simulink model "Smart_City_QCar2_self_driving_stack_r2020a"  (R2020a)
settings: Solver=ode1  StartTime=0.0  StopTime=inf  FixedStep=Controller_Sample_Time  RelTol=1e-3  EnableMultiTasking=on
undefined symbols (not defined in the file): angles_qcar2, Audio_Sample_Time, cal_pos, cameraStepSize, Cobra_Start, Controller_Sample_Time, CSI_Sample_Time, DiscIntNeverNeededParam, engine, gcbh, GyroKF_P0, GyroKF_Q, GyroKF_R, GyroKF_X0, height, HIL, honk, ImageDisplay_Sample_Time, Initialization_Time, Joystick_Sample_Time, JPEG, left, LiDAR_Sample_Time, map_mask, NN_Sample_Time, path_x, path_x2, path_x3, path_x4, path_x5, path_x6, path_x7, path_y, path_y2, path_y3, path_y4, path_y5, path_y6, path_y7, Point, put_me_down, qc_get_step_size, qcar2_lidar_to_map_rotation, QCarEKF_L, QCarEKF_P0, QCarEKF_Q, QCarEKF_R_combined, QCarEKF_R_heading, QcarKF_X0, range_qcar2, RealSense_Sample_Time, top, truck_start, video_display_show, width
libraries: quarc_library x65, simulink_extras x12, simulink x8
(part 2 of 4)

== system Smart_City_QCar2_self_driving_stack_r2020a/Rate Timing Plots/monitorTiming1 ==
  note: moniorTiming Module:
      |
      | This subsystem outputs the sample time and computation time of the model.
      |
      | Outputs:
      | sampleTime (s) n/a : Sample time (unfiltered and filtered) in seconds.
      | computationTime (s) n/a : Computation time (unfiltered and filtered) in seconds.
      |
      | Usage:
      | Compare the Sample Time (s) output to a constant (qc_get_step_size) to monitor whether or not the desired sample time is being achieved. The Computation Time (s) values should be lower than the corresponding sample time value to ensure that the solver has enough time per time step.
  note: Timing Performance
  Computation Time : quarc_library/Sources/Time/Computation Time  sample_time=qc_get_step_size  use_model=on  use_cpu_time=off
  Constant : Constant  Value=qc_get_step_size  SampleTime=-1
  Mux : Mux  Inputs=3
  Sample Time : quarc_library/Sources/Time/Sample Time  Priority=-99  sample_time=qc_get_step_size
  Timing (s) : Outport  VectorParamsAs1DForOutWhenUnconnected=off
  wires:
  Constant/1 -> Mux/2
  Sample Time/1 -> Mux/1
  Mux/1 -> Timing (s)/1
  Computation Time/1 -> Mux/3

== system Smart_City_QCar2_self_driving_stack_r2020a/Rate Timing Plots/monitorTiming2 ==
  note: moniorTiming Module:
      |
      | This subsystem outputs the sample time and computation time of the model.
      |
      | Outputs:
      | sampleTime (s) n/a : Sample time (unfiltered and filtered) in seconds.
      | computationTime (s) n/a : Computation time (unfiltered and filtered) in seconds.
      |
      | Usage:
      | Compare the Sample Time (s) output to a constant (qc_get_step_size) to monitor whether or not the desired sample time is being achieved. The Computation Time (s) values should be lower than the corresponding sample time value to ensure that the solver has enough time per time step.
  note: Timing Performance
  Computation Time : quarc_library/Sources/Time/Computation Time  sample_time=RealSense_Sample_Time  use_model=on  use_cpu_time=off
  Constant : Constant  Value=RealSense_Sample_Time  SampleTime=-1
  Mux : Mux  Inputs=3
  Sample Time : quarc_library/Sources/Time/Sample Time  Priority=-99  sample_time=RealSense_Sample_Time
  Timing (s) : Outport  VectorParamsAs1DForOutWhenUnconnected=off
  wires:
  Constant/1 -> Mux/2
  Sample Time/1 -> Mux/1
  Mux/1 -> Timing (s)/1
  Computation Time/1 -> Mux/3

== system Smart_City_QCar2_self_driving_stack_r2020a/Rate Timing Plots/monitorTiming3 ==
  note: Timing Performance
  note: moniorTiming Module:
      |
      | This subsystem outputs the sample time and computation time of the model.
      |
      | Outputs:
      | sampleTime (s) n/a : Sample time (unfiltered and filtered) in seconds.
      | computationTime (s) n/a : Computation time (unfiltered and filtered) in seconds.
      |
      | Usage:
      | Compare the Sample Time (s) output to a constant (qc_get_step_size) to monitor whether or not the desired sample time is being achieved. The Computation Time (s) values should be lower than the corresponding sample time value to ensure that the solver has enough time per time step.
  Computation Time : quarc_library/Sources/Time/Computation Time  sample_time=ImageDisplay_Sample_Time  use_model=on  use_cpu_time=off
  Constant : Constant  Value=ImageDisplay_Sample_Time  SampleTime=-1
  Mux : Mux  Inputs=3
  Sample Time : quarc_library/Sources/Time/Sample Time  Priority=-99  sample_time=ImageDisplay_Sample_Time
  Timing (s) : Outport  VectorParamsAs1DForOutWhenUnconnected=off
  wires:
  Computation Time/1 -> Mux/3
  Mux/1 -> Timing (s)/1
  Sample Time/1 -> Mux/1
  Constant/1 -> Mux/2

== system Smart_City_QCar2_self_driving_stack_r2020a/Rate Timing Plots/monitorTiming4 ==
  note: Timing Performance
  note: moniorTiming Module:
      |
      | This subsystem outputs the sample time and computation time of the model.
      |
      | Outputs:
      | sampleTime (s) n/a : Sample time (unfiltered and filtered) in seconds.
      | computationTime (s) n/a : Computation time (unfiltered and filtered) in seconds.
      |
      | Usage:
      | Compare the Sample Time (s) output to a constant (qc_get_step_size) to monitor whether or not the desired sample time is being achieved. The Computation Time (s) values should be lower than the corresponding sample time value to ensure that the solver has enough time per time step.
  Computation Time : quarc_library/Sources/Time/Computation Time  sample_time=Joystick_Sample_Time  use_model=on  use_cpu_time=off
  Constant : Constant  Value=Joystick_Sample_Time  SampleTime=-1
  Mux : Mux  Inputs=3
  Sample Time : quarc_library/Sources/Time/Sample Time  Priority=-99  sample_time=Joystick_Sample_Time
  Timing (s) : Outport  VectorParamsAs1DForOutWhenUnconnected=off
  wires:
  Computation Time/1 -> Mux/3
  Mux/1 -> Timing (s)/1
  Sample Time/1 -> Mux/1
  Constant/1 -> Mux/2

== system Smart_City_QCar2_self_driving_stack_r2020a/Rate Timing Plots/monitorTiming5 ==
  note: moniorTiming Module:
      |
      | This subsystem outputs the sample time and computation time of the model.
      |
      | Outputs:
      | sampleTime (s) n/a : Sample time (unfiltered and filtered) in seconds.
      | computationTime (s) n/a : Computation time (unfiltered and filtered) in seconds.
      |
      | Usage:
      | Compare the Sample Time (s) output to a constant (qc_get_step_size) to monitor whether or not the desired sample time is being achieved. The Computation Time (s) values should be lower than the corresponding sample time value to ensure that the solver has enough time per time step.
  note: Timing Performance
  Computation Time : quarc_library/Sources/Time/Computation Time  sample_time=LiDAR_Sample_Time  use_model=on  use_cpu_time=off
  Constant : Constant  Value=LiDAR_Sample_Time  SampleTime=-1
  Mux : Mux  Inputs=3
  Sample Time : quarc_library/Sources/Time/Sample Time  Priority=-99  sample_time=LiDAR_Sample_Time
  Timing (s) : Outport  VectorParamsAs1DForOutWhenUnconnected=off
  wires:
  Constant/1 -> Mux/2
  Sample Time/1 -> Mux/1
  Mux/1 -> Timing (s)/1
  Computation Time/1 -> Mux/3

== system Smart_City_QCar2_self_driving_stack_r2020a/Rate Timing Plots/monitorTiming6 ==
  note: Timing Performance
  note: moniorTiming Module:
      |
      | This subsystem outputs the sample time and computation time of the model.
      |
      | Outputs:
      | sampleTime (s) n/a : Sample time (unfiltered and filtered) in seconds.
      | computationTime (s) n/a : Computation time (unfiltered and filtered) in seconds.
      |
      | Usage:
      | Compare the Sample Time (s) output to a constant (qc_get_step_size) to monitor whether or not the desired sample time is being achieved. The Computation Time (s) values should be lower than the corresponding sample time value to ensure that the solver has enough time per time step.
  Computation Time : quarc_library/Sources/Time/Computation Time  sample_time=NN_Sample_Time  use_model=on  use_cpu_time=off
  Constant : Constant  Value=NN_Sample_Time  SampleTime=-1
  Mux : Mux  Inputs=3
  Sample Time : quarc_library/Sources/Time/Sample Time  Priority=-99  sample_time=NN_Sample_Time
  Timing (s) : Outport  VectorParamsAs1DForOutWhenUnconnected=off
  wires:
  Computation Time/1 -> Mux/3
  Mux/1 -> Timing (s)/1
  Sample Time/1 -> Mux/1
  Constant/1 -> Mux/2

== system Smart_City_QCar2_self_driving_stack_r2020a/Rate Timing Plots/monitorTiming7 ==
  note: Timing Performance
  note: moniorTiming Module:
      |
      | This subsystem outputs the sample time and computation time of the model.
      |
      | Outputs:
      | sampleTime (s) n/a : Sample time (unfiltered and filtered) in seconds.
      | computationTime (s) n/a : Computation time (unfiltered and filtered) in seconds.
      |
      | Usage:
      | Compare the Sample Time (s) output to a constant (qc_get_step_size) to monitor whether or not the desired sample time is being achieved. The Computation Time (s) values should be lower than the corresponding sample time value to ensure that the solver has enough time per time step.
  Computation Time : quarc_library/Sources/Time/Computation Time  sample_time=1  use_model=on  use_cpu_time=off
  Constant : Constant  SampleTime=-1
  Mux : Mux  Inputs=3
  Sample Time : quarc_library/Sources/Time/Sample Time  Priority=-99  sample_time=1
  Timing (s) : Outport  VectorParamsAs1DForOutWhenUnconnected=off
  wires:
  Computation Time/1 -> Mux/3
  Mux/1 -> Timing (s)/1
  Sample Time/1 -> Mux/1
  Constant/1 -> Mux/2

== system Smart_City_QCar2_self_driving_stack_r2020a/Rate Timing Plots/monitorTiming8 ==
  note: moniorTiming Module:
      |
      | This subsystem outputs the sample time and computation time of the model.
      |
      | Outputs:
      | sampleTime (s) n/a : Sample time (unfiltered and filtered) in seconds.
      | computationTime (s) n/a : Computation time (unfiltered and filtered) in seconds.
      |
      | Usage:
      | Compare the Sample Time (s) output to a constant (qc_get_step_size) to monitor whether or not the desired sample time is being achieved. The Computation Time (s) values should be lower than the corresponding sample time value to ensure that the solver has enough time per time step.
  note: Timing Performance
  Computation Time : quarc_library/Sources/Time/Computation Time  sample_time=Audio_Sample_Time  use_model=on  use_cpu_time=off
  Constant : Constant  Value=Audio_Sample_Time  SampleTime=-1
  Mux : Mux  Inputs=3
  Sample Time : quarc_library/Sources/Time/Sample Time  Priority=-99  sample_time=Audio_Sample_Time
  Timing (s) : Outport  VectorParamsAs1DForOutWhenUnconnected=off
  wires:
  Constant/1 -> Mux/2
  Sample Time/1 -> Mux/1
  Mux/1 -> Timing (s)/1
  Computation Time/1 -> Mux/3

== system Smart_City_QCar2_self_driving_stack_r2020a/RealSense Camera/Newer Depth ==
  In1 : Inport
  Channel : quarc_library/Signal Routing/Channel  channel=0  buffer_size=1
  Image Compress : quarc_library/Image Processing/Generic/Image Compress  algorithm=JPEG  source=Internal dialog parameter  quality=quality  output_dim=-1
  Video Display : quarc_library/Multimedia/Video Display  Tag=Smart_City_QCar2_self_driving_stack_r2020a/RealSense Camera/Newer Depth/Video Display  sample_time=sample_time  use_hardware=on
  wires:
  Image Compress/1 -> Channel/1
  In1/1 -> Image Compress/1
  Channel/1 -> Video Display/1

== system Smart_City_QCar2_self_driving_stack_r2020a/RealSense Camera/RealSense Capture ==
  AND : Logic  Commented=on  AllPortsSameDT=off  OutDataTypeStr=boolean
  AND1 : Logic  Commented=on  IconShape=distinctive  AllPortsSameDT=off  OutDataTypeStr=boolean
  Compare To Constant : simulink/Logic and Bit Operations/Compare To Constant  Commented=on  relop===  const=2  OutDataTypeStr=boolean
  Compare To Constant1 : simulink/Logic and Bit Operations/Compare To Constant  Commented=on  relop=>=  const=0  OutDataTypeStr=boolean
  Constant : Constant  Commented=on  Value=[1 0 0 0 0]
  Display : Display  Commented=on
  Display1 : Display  Commented=on
  Display2 : Display  Commented=on
  Image Compress : quarc_library/Image Processing/Generic/Image Compress  Commented=on  algorithm=JPEG  source=Internal dialog parameter  quality=50  output_dim=-1
  Image Filter : quarc_library/Image Processing/Generic/Image Filter  filter_type=Depth hole-fill  source_of_roi=Internal dialog parameter  roi_style=[top, left, height, width]  roi=[]  maximum_roi=[]  roi_zone=Operate inside region of interest  border_type=Replicate  border_value=[0 0 0]  kernel_size=5  sigma=10  mask_size=[3 3]  kernel=int16([-2 -1 0; -1 1 1; 0 1 2])  divisor=1  offset=0  rounding=Nearest  algorithm_hint=None  threshold=100  alpha=0.9  num_frames=8  num_valid=1  gap_threshold=10  depth_threshold=255  iterations=2  norm_type=L1
      settings: AttributesFormatString=(%<filter_type>)  SourceProductName=QUARC Targets
  Image Filter1 : quarc_library/Image Processing/Generic/Image Filter  filter_type=Depth temporal low-pass  source_of_roi=Internal dialog parameter  roi_style=[top, left, height, width]  roi=[]  maximum_roi=[]  roi_zone=Operate inside region of interest  border_type=Replicate  border_value=[0 0 0]  kernel_size=5  sigma=10  mask_size=[3 3]  kernel=int16([-2 -1 0; -1 1 1; 0 1 2])  divisor=1  offset=0  rounding=Nearest  algorithm_hint=None  threshold=100  alpha=0.9  num_frames=4  num_valid=1  gap_threshold=10  depth_threshold=255  iterations=2  norm_type=L1
      settings: AttributesFormatString=(%<filter_type>)  SourceProductName=QUARC Targets
  Memory : Memory  Commented=on  InheritSampleTime=on
  NN New : Scope  Commented=on
  NN Receive : Scope  Commented=on
  Rate Transition : RateTransition  Commented=on  OutPortSampleTime=NN_Sample_Time
  Scope : Scope
  Stream Server : quarc_library/Communications/Basic/Stream Server  Commented=on  uri_source=Specify via dialog (do not evaluate)  uri=tcpip://remotehost:18999  send_buffer_size=640*360*3  receive_buffer_size=6*32  byte_order=little endian (Intel - LSB first)  optimization=Minimum latency  send_options=Send most recent data  receive_options=Receive most recent data  default_value=zeros(1,5,'single')  sample_time=NN_Sample_Time  active=off  implementation=Use blocking I/O in a separate thread  send_fifo_size=2  receive_fifo_size=2  send_priority=0  receive_priority=0  send_dimensions=on  receive_dimensions=off  max_dimensions=-1  data_type=single  type_expr=BusObject
      settings: AttributesFormatString="\"tcpip://remotehost:18999\""
  Switch : Switch  Commented=on  Criteria=u2 > Threshold  Threshold=0.5
  Terminator{,1..4} (5 alike) : Terminator
  Terminator5 : Terminator  Commented=on
  Video3D Capture : quarc_library/Multimedia/Video3D Capture  object_name=RealSense  stream_type=Depth  stream_index=0  resolution=640 x 360  width=640  height=360  output_format=Distance in meters (HxW)  data_type=single  sample_time=RealSense_Sample_Time  camera_intrinsics=off  depth_scale=off  brightness_override=Do not override  brightness=50.0  contrast_override=Do not override  contrast=50.0  hue_override=Do not override  hue=50.0  saturation_override=Do not override  saturation=50.0  sharpness_override=Do not override  sharpness=50.0  gamma_override=Do not override  gamma=50.0  gain_override=Do not override  gain=50.0  backlightcompensation_override=Do not override  backlightcompensation=50.0  whitebalance_override=Automatic white balance  whitebalance=50.0  exposure_override=Automatic exposure  exposure=30.0  emitter=Enable laser emitter  preset=Do not set camera presets
  Video3D Capture1 : quarc_library/Multimedia/Video3D Capture  object_name=RealSense  stream_type=RGB  stream_index=0  resolution=1920 x 1080  width=1920  height=1080  output_format=MATLAB RGB (HxWx3)  data_type=uint8  sample_time=RealSense_Sample_Time*1  camera_intrinsics=off  depth_scale=off  brightness_override=Do not override  brightness=50.0  contrast_override=Do not override  contrast=50.0  hue_override=Do not override  hue=50.0  saturation_override=Do not override  saturation=50.0  sharpness_override=Do not override  sharpness=50.0  gamma_override=Do not override  gamma=50.0  gain_override=Do not override  gain=50.0  backlightcompensation_override=Do not override  backlightcompensation=50.0  whitebalance_override=Automatic white balance  whitebalance=50.0  exposure_override=Automatic exposure  exposure=30.0  emitter=Enable laser emitter  preset=Do not set camera presets
  Video3D Initialize : quarc_library/Multimedia/Video3D Initialize  object_name=RealSense  source=Device  identifier=0  file=sample.bag  sample_time=RealSense_Sample_Time  active=on
  New : Outport
  Depth Image : Outport  Port=2
  Sign Probabilities : Outport  Port=3
  wires:
  Video3D Capture/4 -> New/1
  Video3D Capture/2 -> Terminator4/1
  Video3D Capture/3 -> Terminator3/1
  Video3D Capture/1 -> Image Filter/1
  Video3D Initialize/1 -> Terminator/1
  Switch/1 -> Sign Probabilities/1
  Video3D Capture1/1 -> Rate Transition/1
  Constant/1 -> Switch/3
  Compare To Constant1/1 -> AND/2
  Stream Server/4 -> NN Receive/1, Switch/1
  Stream Server/2 -> Compare To Constant1/1, Display1/1
  Stream Server/5 -> NN New/1, Switch/2
  Stream Server/3 -> Terminator5/1
  Compare To Constant/1 -> AND/1
  Video3D Capture1/2 -> Terminator1/1
  Video3D Capture1/3 -> Terminator2/1
  Stream Server/1 -> Compare To Constant/1, Display/1
  Memory/1 -> AND1/2
  AND/1 -> Display2/1, Memory/1
  Video3D Capture1/4 -> Scope/1, AND1/1
  AND1/1 -> Stream Server/2
  Rate Transition/1 -> Image Compress/1
  Image Compress/1 -> Stream Server/1
  Image Filter/1 -> Image Filter1/1
  Image Filter1/1 -> Depth Image/1

== system Smart_City_QCar2_self_driving_stack_r2020a/RealSense Camera/obstacleDetection Markham March 22 ==
  note: %
  note: m
  note: m
  note: %
  note: px
  note: px
  note: %
  note: %
  imageDepth : Inport
  steering (rad) : Inport  Port=2
  Enable : EnablePort  PropagateVarSize=During execution
  Add : Sum
  Bias : Constant  Value=0
  Box Color : Constant  Value=[255 0 0]
  Constant1 : Constant  Value=200
  Constant2 : Constant  Value=.15
  Constant3 : Constant
  Constant4 : Constant  Value=50
  Constant5 : Constant  Value=0.5
  Constant6 : Constant  Value=0.5
  Constant7 : Constant  Value=0.6
  Constant8 : Constant  Value=0.6
  Display : Display
  Draw Lines Module : MATLAB Function  TreatAsAtomicUnit=on
  Image Convert : quarc_library/Image Processing/Generic/Image Convert  input_format=MATLAB greyscale (HxW)  padding=0  output_format=MATLAB greyscale (HxW)  data_type=uint16
      settings: AttributesFormatString=(%<input_format>)  SourceProductName=QUARC Targets
  Saturation : Saturate  UpperLimit=2  LowerLimit=0.05
  Saturation1 : Saturate  UpperLimit=1  LowerLimit=0
  Scope : Scope
  Steering based image subselector : MATLAB Function  TreatAsAtomicUnit=on
  max white for 8m : Gain  Gain=1/2.5
  imageDepthForDisplay : Outport  VectorParamsAs1DForOutWhenUnconnected=off
  distance (m) : Outport  Port=2  VectorParamsAs1DForOutWhenUnconnected=off
  wires:
  Saturation1/1 -> Image Convert/1
  Constant6/1 -> Steering based image subselector/8(maxSteering)
  Steering based image subselector/2(distance) -> Add/1, Scope/1
  Constant5/1 -> Steering based image subselector/7(vertCenter)
  Constant4/1 -> Steering based image subselector/6(height)
  Constant1/1 -> Steering based image subselector/5(width)
  Constant3/1 -> Steering based image subselector/4(maxDistance)
  Constant2/1 -> Steering based image subselector/3(minDistance)
  steering (rad)/1 -> Steering based image subselector/2(steering)
  Draw Lines Module/1(img_out) -> imageDepthForDisplay/1
  Steering based image subselector/1(pts) -> Draw Lines Module/2(pts)
  Image Convert/1 -> Draw Lines Module/1(img_in)
  max white for 8m/1 -> Saturation1/1
  imageDepth/1 -> Steering based image subselector/1(depth), max white for 8m/1
  Bias/1 -> Add/2
  Add/1 -> Saturation/1, Display/1
  Saturation/1 -> distance (m)/1
  Box Color/1 -> Draw Lines Module/3(color)
  Constant7/1 -> Steering based image subselector/9(reduction)
  Constant8/1 -> Steering based image subselector/10(maxSteeringWidth)

== system Smart_City_QCar2_self_driving_stack_r2020a/Speed & Steering Commander/Cross Track Controller ==
  closest point : Inport
  distance : Inport  Port=2
  xy : Inport  Port=3
  Heading : Inport  Port=4
  Commanded_Speed : Inport  Port=5
  Path : Inport  Port=6
  Constant : Constant  Value=0
  Constant1 : Constant
  Constant6 : Constant  Value=Initialization_Time
  Cos : Trigonometry  Operator=cos
  Cos1 : Trigonometry
  Cross Product : quarc_library/Math Operations/Vectors/Cross Product
      settings: SourceProductName=QUARC Targets
  Demux : Demux  Outputs=3
  Equal : RelationalOperator  Operator===  OutDataTypeStr=boolean  RndMeth=Simplest
  Equal1 : RelationalOperator  Operator=~=  OutDataTypeStr=boolean  RndMeth=Simplest
  Gain3 : Gain
  Gain6 : Gain  Gain=3
  GreaterThan : RelationalOperator  Operator=<  OutDataTypeStr=boolean  RndMeth=Simplest
  Integrator : Integrator  ExternalReset=level  LimitOutput=on  UpperSaturationLimit=.2  LowerSaturationLimit=-.2
  Integrator1 : Integrator  ExternalReset=level  LimitOutput=on  UpperSaturationLimit=1  LowerSaturationLimit=0
  Memory1 : Memory  InitialCondition=6  InheritSampleTime=on  LinearizeMemory=on  LinearizeAsDelay=on
  Mux : Mux  Inputs=3
  Mux1 : Mux  Inputs=2
  Mux2 : Mux  Inputs=2
  OR : Logic  Operator=OR  Inputs=3  IconShape=distinctive  AllPortsSameDT=off  OutDataTypeStr=boolean
  Product : Product
  Product3 : Product
  Radians to Degrees : simulink_extras/Transformations/Radians to Degrees
  Saturation1 : Saturate  UpperLimit=.2  LowerLimit=-.2
  Scope1 : Scope  NumInputPorts=2
  Sign : Signum
  Sum : Sum  Inputs=+-
  Sum2 : Sum
  Time1 : quarc_library/Sources/Time/Time  time_source=Wall clock  sample_time=qc_get_step_size
  steering correction : Outport
  wires:
  Heading/1 -> Cos1/1, Cos/1
  Cos/1 -> Mux/1
  Cos1/1 -> Mux/2
  xy/1 -> Sum/2
  closest point/1 -> Sum/1
  Sum/1 -> Mux1/1
  Mux1/1 -> Cross Product/2
  Mux/1 -> Cross Product/1
  Cross Product/1 -> Demux/1
  Demux/3 -> Sign/1
  Sign/1 -> Product3/1
  Gain6/1 -> Integrator/1
  Product3/1 -> Gain3/1, Gain6/1
  Integrator/1 -> Mux2/1, Sum2/1
  Saturation1/1 -> Mux2/2, Sum2/2
  distance/1 -> Product3/2
  Sum2/1 -> steering correction/1
  Commanded_Speed/1 -> Equal/1
  Constant/1 -> Equal/2
  Path/1 -> Equal1/2, Memory1/1
  Memory1/1 -> Equal1/1
  Equal1/1 -> OR/2
  Equal/1 -> OR/1
  OR/1 -> Scope1/1, Integrator1/2, Integrator/2
  Constant1/1 -> Integrator1/1
  Product/1 -> Saturation1/1
  Gain3/1 -> Product/1
  Integrator1/1 -> Product/2
  Mux2/1 -> Radians to Degrees/1
  Radians to Degrees/1 -> Scope1/2
  Time1/1 -> GreaterThan/1
  Constant6/1 -> GreaterThan/2
  GreaterThan/1 -> OR/3

== system Smart_City_QCar2_self_driving_stack_r2020a/Speed & Steering Commander/Infrastructure Car Detection Speed Adjust ==
  obstacleDistance (m) : Inport
  Desired Speed Command : Inport  Port=2
  Constant : Constant  Value=0.3
  Constant1 : Constant  Value=.4
  Constant2 : Constant
  Less Than : RelationalOperator  Operator=<  OutDataTypeStr=boolean  RndMeth=Simplest
  MATLAB Function : MATLAB Function  TreatAsAtomicUnit=on
  Scope : Scope  NumInputPorts=2
  Adjusted Speed Command : Outport  VectorParamsAs1DForOutWhenUnconnected=off
  Honk : Outport  Port=2
  wires:
  Desired Speed Command/1 -> MATLAB Function/4(nominal_speed)
  MATLAB Function/1(speed_cmd) -> Adjusted Speed Command/1, Scope/1
  Less Than/1 -> Honk/1
  Constant1/1 -> Less Than/2
  obstacleDistance (m)/1 -> MATLAB Function/1(obstacle_distance), Scope/2, Less Than/1
  Constant/1 -> MATLAB Function/2(stop_distance)  "stop distance (m)"
  Constant2/1 -> MATLAB Function/3(nominal_tracking_distance)  "nominal tracking distance (m)"

== system Smart_City_QCar2_self_driving_stack_r2020a/Speed & Steering Commander/Path Commander ==
  note: Tunable
      | Params
  note: Changed the abs and the duration
  path : Inport
  xy : Inport  Port=2
  look_ahead_d : Inport  Port=3
  Data Type Conversion : DataTypeConversion
  Display : Display
  "Distance  " : Scope
  Distance (m) to a viable path : Constant  Value=0.05
  Duration that car is within distance of viable path : Constant  Value=0.2
  Less Than Threshold : Subsystem
  Multiport Switch : MultiPortSwitch  Inputs=7  DiagnosticForDefault=None
  Multiport Switch1 : MultiPortSwitch  Inputs=7  DiagnosticForDefault=None
  Multiport Switch2 : MultiPortSwitch  Inputs=7  DiagnosticForDefault=None
  Mux : Mux  Inputs=7
  Path 1  Look Ahead Generator : Subsystem
  Path 2  Look Ahead Generator : Subsystem
  Path 3  Look Ahead Generator : Subsystem
  Path 4  Look Ahead Generator : Subsystem
  Path 5  Look Ahead Generator : Subsystem
  Path 6  Look Ahead Generator : Subsystem
  Path 7  Look Ahead Generator : Subsystem
  Turn Paths on and Off : Gain  Gain=map_mask
  xy_cmd : Outport
  Path_Options : Outport  Port=2
  closest point : Outport  Port=3
  distance : Outport  Port=4
  wires:
  look_ahead_d/1 -> Path 7  Look Ahead Generator/2(look_ahead_d), Path 6  Look Ahead Generator/2(look_ahead_d), Path 5  Look Ahead Generator/2(look_ahead_d), Path 4  Look Ahead Generator/2(look_ahead_d), Path 3  Look Ahead Generator/2(look_ahead_d), Path 2  Look Ahead Generator/2(look_ahead_d), Path 1  Look Ahead Generator/2(look_ahead_d)
  path/1 -> Multiport Switch2/1, Multiport Switch1/1, Multiport Switch/1
  Path 1  Look Ahead Generator/1(xy_cmd) -> Multiport Switch/2
  Path 2  Look Ahead Generator/1(xy_cmd) -> Multiport Switch/3
  Multiport Switch/1 -> xy_cmd/1
  Path 3  Look Ahead Generator/1(xy_cmd) -> Multiport Switch/4
  Path 4  Look Ahead Generator/1(xy_cmd) -> Multiport Switch/5
  Path 1  Look Ahead Generator/3(distance) -> Multiport Switch2/2, Mux/1
  Path 2  Look Ahead Generator/3(distance) -> Multiport Switch2/3, Mux/2
  Path 3  Look Ahead Generator/3(distance) -> Multiport Switch2/4, Mux/3
  Path 4  Look Ahead Generator/3(distance) -> Multiport Switch2/5, Mux/4
  Mux/1 -> "Distance  "/1, Less Than Threshold/1(Distances)
  Distance (m) to a viable path/1 -> Less Than Threshold/2(Distance Threshold)
  Duration that car is within distance of viable path/1 -> Less Than Threshold/3(Duration Threshold)
  Less Than Threshold/1(elapsed) -> Data Type Conversion/1, Display/1
  Turn Paths on and Off/1 -> Path_Options/1
  Data Type Conversion/1 -> Turn Paths on and Off/1
  Path 5  Look Ahead Generator/1(xy_cmd) -> Multiport Switch/6
  Path 6  Look Ahead Generator/1(xy_cmd) -> Multiport Switch/7
  Path 5  Look Ahead Generator/3(distance) -> Multiport Switch2/6, Mux/5
  Path 6  Look Ahead Generator/3(distance) -> Multiport Switch2/7, Mux/6
  Path 1  Look Ahead Generator/2(closest_point) -> Multiport Switch1/2
  Path 2  Look Ahead Generator/2(closest_point) -> Multiport Switch1/3
  Path 3  Look Ahead Generator/2(closest_point) -> Multiport Switch1/4
  Path 4  Look Ahead Generator/2(closest_point) -> Multiport Switch1/5
  Path 5  Look Ahead Generator/2(closest_point) -> Multiport Switch1/6
  Path 6  Look Ahead Generator/2(closest_point) -> Multiport Switch1/7
  Multiport Switch1/1 -> closest point/1
  Multiport Switch2/1 -> distance/1
  xy/1 -> Path 7  Look Ahead Generator/1(xy), Path 6  Look Ahead Generator/1(xy), Path 5  Look Ahead Generator/1(xy), Path 4  Look Ahead Generator/1(xy), Path 3  Look Ahead Generator/1(xy), Path 2  Look Ahead Generator/1(xy), Path 1  Look Ahead Generator/1(xy)
  Path 7  Look Ahead Generator/1(xy_cmd) -> Multiport Switch/8
  Path 7  Look Ahead Generator/2(closest_point) -> Multiport Switch1/8
  Path 7  Look Ahead Generator/3(distance) -> Mux/7, Multiport Switch2/8

== system Smart_City_QCar2_self_driving_stack_r2020a/Speed & Steering Commander/Realsense Obstacle Detection Speed Adjust ==
  obstacleDistance (m) : Inport
  Desired Speed Command : Inport  Port=2
  Constant : Constant  Value=0.375
  Constant1 : Constant  Value=.4
  Constant2 : Constant  Value=0.6
  Less Than : RelationalOperator  Operator=<  OutDataTypeStr=boolean  RndMeth=Simplest
  MATLAB Function : MATLAB Function  TreatAsAtomicUnit=on
  Scope : Scope  NumInputPorts=2
  Adjusted Speed Command : Outport  VectorParamsAs1DForOutWhenUnconnected=off
  Honk : Outport  Port=2
  wires:
  Constant2/1 -> MATLAB Function/3(nominal_tracking_distance)  "nominal tracking distance (m)"
  Constant/1 -> MATLAB Function/2(stop_distance)  "stop distance (m)"
  obstacleDistance (m)/1 -> Less Than/1, Scope/2, MATLAB Function/1(obstacle_distance)
  Constant1/1 -> Less Than/2
  Less Than/1 -> Honk/1
  MATLAB Function/1(speed_cmd) -> Scope/1, Adjusted Speed Command/1
  Desired Speed Command/1 -> MATLAB Function/4(nominal_speed)

== system Smart_City_QCar2_self_driving_stack_r2020a/Speed & Steering Commander/Sign Finder ==
  Signs : Inport
  Constant1 : Constant  Value=.8
  Constant15 : Constant  Value=.9
  Constant16 : Constant  Value=.06
  Constant2 : Constant  Value=.06
  Demux : Demux  Outputs=5
  Greater Than Threshold : Subsystem
  Greater Than Threshold1 : Subsystem
  Stop Sign : Outport
  Slow Sign : Outport  Port=2
  wires:
  Signs/1 -> Demux/1
  Constant16/1 -> Greater Than Threshold/3(Duration)
  Constant15/1 -> Greater Than Threshold/2(Threshold)
  Demux/4 -> Greater Than Threshold/1(Signal)
  Greater Than Threshold/1(elapsed) -> Stop Sign/1
  Greater Than Threshold1/1(elapsed) -> Slow Sign/1
  Demux/3 -> Greater Than Threshold1/1(Signal)
  Constant1/1 -> Greater Than Threshold1/2(Threshold)
  Constant2/1 -> Greater Than Threshold1/3(Duration)

== system Smart_City_QCar2_self_driving_stack_r2020a/Speed & Steering Commander/Steering Based on LiDAR ==
  xy_command : Inport
  xy : Inport  Port=2
  heading : Inport  Port=3
  Direction Vector Generator : Subsystem
  Display1 : Display
      settings: Decimation=100
  Gain1 : Gain
  Radians to Degrees1 : simulink_extras/Transformations/Radians to Degrees
  Steering Commander : MATLAB Function  TreatAsAtomicUnit=on
  distance : Outport
  LiDAR Steering : Outport  Port=2
  wires:
  Direction Vector Generator/1(distance) -> distance/1
  xy_command/1 -> Direction Vector Generator/1(xy_command)
  Direction Vector Generator/2(aoa) -> Radians to Degrees1/1, Steering Commander/1(aoa)
  Gain1/1 -> LiDAR Steering/1
  Radians to Degrees1/1 -> Display1/1
  xy/1 -> Direction Vector Generator/2(xy)
  heading/1 -> Direction Vector Generator/3(heading)
  Steering Commander/1(steering) -> Gain1/1

== system Smart_City_QCar2_self_driving_stack_r2020a/Speed & Steering Commander/Traffic Zone 1 ==
  note: [1 -.3] %[1,5 0]
  note: [0.2 -0.7]
  note: select the control variable
  xy : Inport
  speed in : Inport  Port=2
  Traffic Light : Inport  Port=3
  AND : Logic  Inputs=4  IconShape=distinctive  AllPortsSameDT=off  OutDataTypeStr=boolean
  Bias : Bias  Bias=-0.4
  Constant13 : Constant  Value=[-0.61 -1.21]
  Constant14 : Constant  Value=[-0.4 -0.86]
  Constant3 : Constant  Value=.1
  Demux : Demux  Outputs=2
  Demux1 : Demux  Outputs=2
  Demux2 : Demux  Outputs=2
  Display : Display
  Gain : Gain
  Greater Than Threshold : Subsystem
  Less Than Threshold : Subsystem
  MATLAB Function2 : MATLAB Function  TreatAsAtomicUnit=on
  Memory7 : Memory  InitialCondition=1  InheritSampleTime=on  LinearizeMemory=on  LinearizeAsDelay=on
  Saturation : Saturate  UpperLimit=1  LowerLimit=0
  "Speed " : Scope
  Speed Multi : Scope
  Traffic State : Display
  in zone : Display
  Speed Out : Outport
  wires:
  xy/1 -> Greater Than Threshold/1(Signal), Less Than Threshold/1(Signal), Demux2/1
  Constant3/1 -> Less Than Threshold/3(Duration), Greater Than Threshold/3(Duration)
  Constant13/1 -> Greater Than Threshold/2(Threshold)
  Constant14/1 -> Less Than Threshold/2(Threshold)
  Greater Than Threshold/1(elapsed) -> Demux/1
  Demux/2 -> AND/2
  Demux/1 -> AND/1
  Less Than Threshold/1(elapsed) -> Demux1/1
  Demux1/2 -> AND/4
  Demux1/1 -> AND/3
  Demux2/1 -> Bias/1
  Bias/1 -> Gain/1
  Gain/1 -> Saturation/1
  MATLAB Function2/1(Traffic_State) -> Memory7/1, Traffic State/1
  Memory7/1 -> MATLAB Function2/1(Previous_State)
  speed in/1 -> MATLAB Function2/2(Speed_In)
  AND/1 -> MATLAB Function2/4(In_Zone), in zone/1
  Saturation/1 -> Speed Multi/1, MATLAB Function2/3(Speed_Multi)
  MATLAB Function2/2(Speed_Out) -> Speed Out/1, "Speed "/1
  Traffic Light/1 -> Display/1, MATLAB Function2/5(Traffic_Light)  "1 means green"

== system Smart_City_QCar2_self_driving_stack_r2020a/Speed & Steering Commander/Traffic Zone 2 ==
  note: select the control variable
  xy : Inport
  speed in : Inport  Port=2
  Traffic Light : Inport  Port=3
  AND : Logic  Inputs=4  IconShape=distinctive  AllPortsSameDT=off  OutDataTypeStr=boolean
  Bias : Bias  Bias=0.8
  Constant13 : Constant  Value=[0.75 -0.9]
  Constant14 : Constant  Value=[1.35 -0.65]
  Constant3 : Constant  Value=.1
  Demux : Demux  Outputs=2
  Demux1 : Demux  Outputs=2
  Demux2 : Demux  Outputs=2
  Display : Display
  Gain : Gain  Gain=-1
  Greater Than Threshold : Subsystem
  Less Than Threshold : Subsystem
  MATLAB Function2 : MATLAB Function  TreatAsAtomicUnit=on
  Memory7 : Memory  InitialCondition=1  InheritSampleTime=on  LinearizeMemory=on  LinearizeAsDelay=on
  Saturation : Saturate  UpperLimit=1  LowerLimit=0
  "Speed " : Scope
  Speed Multi : Scope
  Traffic State : Display
  in zone : Display
  Speed Out : Outport
  wires:
  MATLAB Function2/2(Speed_Out) -> "Speed "/1, Speed Out/1
  Saturation/1 -> MATLAB Function2/3(Speed_Multi), Speed Multi/1
  AND/1 -> in zone/1, MATLAB Function2/4(In_Zone)
  speed in/1 -> MATLAB Function2/2(Speed_In)
  Memory7/1 -> MATLAB Function2/1(Previous_State)
  MATLAB Function2/1(Traffic_State) -> Traffic State/1, Memory7/1
  Gain/1 -> Saturation/1
  Bias/1 -> Gain/1
  Demux2/1 -> Bias/1
  Demux1/1 -> AND/3
  Demux1/2 -> AND/4
  Less Than Threshold/1(elapsed) -> Demux1/1
  Demux/1 -> AND/1
  Demux/2 -> AND/2
  Greater Than Threshold/1(elapsed) -> Demux/1
  Constant14/1 -> Less Than Threshold/2(Threshold)
  Constant13/1 -> Greater Than Threshold/2(Threshold)
  Constant3/1 -> Greater Than Threshold/3(Duration), Less Than Threshold/3(Duration)
  xy/1 -> Greater Than Threshold/1(Signal), Less Than Threshold/1(Signal), Demux2/1
  Traffic Light/1 -> Display/1, MATLAB Function2/5(Traffic_Light)

== system Smart_City_QCar2_self_driving_stack_r2020a/Speed & Steering Commander/xy signal maker ==
  xy 1 : Inport
  xy 2 : Inport  Port=2
  Demux1 : Demux  Outputs=2
  Demux2 : Demux  Outputs=2
  Mux : Mux  Inputs=2
  Mux1 : Mux  Inputs=2
  Rate Transition1 : RateTransition  OutPortSampleTime=ImageDisplay_Sample_Time
  Rate Transition2 : RateTransition  OutPortSampleTime=ImageDisplay_Sample_Time
  x : Outport
  y : Outport  Port=2
  wires:
  Demux2/1 -> Mux/2
  Demux1/2 -> Mux1/1
  Demux1/1 -> Mux/1
  Demux2/2 -> Mux1/2
  Mux/1 -> x/1
  Mux1/1 -> y/1
  xy 1/1 -> Rate Transition1/1
  Rate Transition1/1 -> Demux1/1
  xy 2/1 -> Rate Transition2/1
  Rate Transition2/1 -> Demux2/1

== system Smart_City_QCar2_self_driving_stack_r2020a/QCar 2/Fusion Comparison & Kalman Estimator/Angle mod1 ==
  Angle : Inport
  Bias : Bias  Bias=180
  Bias1 : Bias  Bias=-180
  Constant1 : Constant  Value=360
  Mod : Math  Operator=mod  SaturateOnIntegerOverflow=on
  Mod_Angle : Outport
  wires:
  Angle/1 -> Bias/1
  Bias1/1 -> Mod_Angle/1
  Bias/1 -> Mod/1
  Constant1/1 -> Mod/2
  Mod/1 -> Bias1/1

== system Smart_City_QCar2_self_driving_stack_r2020a/QCar 2/LiDAR/Match Scans ==
  Current_Distance : Inport
  Angles : Inport  Port=2
  Ref_Distance : Inport  Port=3
  Ref_Angles : Inport  Port=4
  absolute_scan : Inport  Port=5
  Previous Estimate : Inport  Port=6
  Enable : EnablePort  PropagateVarSize=During execution
  # LIDAR Elements : Scope
  Constant : Constant  Value=[8 8 2*pi]
  Constant1 : Constant  Value=[1.5 1.5 pi/2]
  Data Type Conversion : DataTypeConversion
  Data Type Conversion1 : DataTypeConversion
  Demux : Demux  Outputs=2
  Display : Display
  Gain : Gain  Gain=[1 -1 -1]
  Gain1 : Gain  Gain=[1 -1 -1]
  LIDAR Scan Match : quarc_library/Image Processing/Generic/LIDAR Scan Match  mode=Variable-size input  resolution=35  max_range=8  use_initial_pose=on
      settings: SourceProductName=QUARC Targets
  MATLAB Function : MATLAB Function  TreatAsAtomicUnit=on
  Memory : Memory  InitialCondition=[0 0 0]  InheritSampleTime=on  LinearizeMemory=on  LinearizeAsDelay=on
  Pose Deltas : Scope
  Subtract : Sum  Inputs=+-
  Switch : Switch  Criteria=u2 > Threshold  Threshold=.5
  Width : Width
  pose : Outport
  score : Outport  Port=2
  wires:
  LIDAR Scan Match/1 -> Memory/1, Subtract/1, Gain/1  "pose"
  Ref_Distance/1 -> LIDAR Scan Match/3
  Ref_Angles/1 -> LIDAR Scan Match/4
  Gain/1 -> Data Type Conversion/1
  LIDAR Scan Match/2 -> score/1
  Memory/1 -> Subtract/2
  absolute_scan/1 -> Switch/2
  Switch/1 -> Demux/1, Display/1
  Demux/1 -> LIDAR Scan Match/6
  Demux/2 -> LIDAR Scan Match/7
  Constant/1 -> Switch/1
  Constant1/1 -> Switch/3
  Data Type Conversion/1 -> pose/1
  MATLAB Function/1(new_range) -> Width/1, LIDAR Scan Match/1
  MATLAB Function/2(new_angles) -> LIDAR Scan Match/2
  Width/1 -> # LIDAR Elements/1
  Subtract/1 -> Pose Deltas/1
  Previous Estimate/1 -> Data Type Conversion1/1
  Gain1/1 -> LIDAR Scan Match/5
  Data Type Conversion1/1 -> Gain1/1
  Current_Distance/1 -> MATLAB Function/1(range)
  Angles/1 -> MATLAB Function/2(angles)

== system Smart_City_QCar2_self_driving_stack_r2020a/QCar 2/LiDAR/RisingEdge ==
  Input : Inport
  Logical Operator1 : Logic  AllPortsSameDT=off
  Logical Operator2 : Logic  Operator=NOT  AllPortsSameDT=off
  Memory : Memory  InheritSampleTime=on  LinearizeMemory=on
  RisingEdgeTrigger : Outport  VectorParamsAs1DForOutWhenUnconnected=off
  wires:
  Logical Operator1/1 -> RisingEdgeTrigger/1
  Logical Operator2/1 -> Logical Operator1/2
  Memory/1 -> Logical Operator2/1
  Input/1 -> Logical Operator1/1, Memory/1

== system Smart_City_QCar2_self_driving_stack_r2020a/QCar 2/LiDAR/captureLIDAR ==
  Display : Display
      settings: Decimation=100
  Display1 : Display
      settings: Decimation=100
  Display2 : Display
      settings: Decimation=100
  Ranging Sensor : quarc_library/Devices/Third-Party/Sensors/Ranging Sensor  sensor_type=RPLidar LIDAR  uri=serial-cpu://localhost:1?baud='256000',word='8',parity='none',stop='1',flow='none',dsr='on'  ranging_distance=Long  timing_budget=0.033  measurement_period=0.040  output_mode=Variable-size output  samples_per_revolution=SPR_qcar2  max_distance=0.050  max_angle=5  sample_time=LiDAR_Sample_Time  show_versions=on  active=on
      settings: SourceProductName=QUARC Targets
  distances (m) : Outport  VectorParamsAs1DForOutWhenUnconnected=off
  Heading (rad) : Outport  Port=2  VectorParamsAs1DForOutWhenUnconnected=off
  qual : Outport  Port=3  VectorParamsAs1DForOutWhenUnconnected=off
  new : Outport  Port=4  VectorParamsAs1DForOutWhenUnconnected=off
  wires:
  Ranging Sensor/1 -> distances (m)/1
  Ranging Sensor/3 -> Heading (rad)/1
  Ranging Sensor/4 -> qual/1
  Ranging Sensor/5 -> new/1
  Ranging Sensor/6 -> Display/1
  Ranging Sensor/7 -> Display1/1
  Ranging Sensor/8 -> Display2/1

== system Smart_City_QCar2_self_driving_stack_r2020a/QCar 2/LiDAR/rising edge latch ==
  rising edge trigger : Inport
  input : Inport  Port=2
  untriggered output : Inport  Port=3
  Latch Input : Subsystem  TreatAsAtomicUnit=on
  Switch : Switch  Threshold=0.5
  output : Outport  VectorParamsAs1DForOutWhenUnconnected=off
  wires:
  untriggered output/1 -> Switch/3
  Switch/1 -> output/1
  Latch Input/1(Latch) -> Switch/1
  Latch Input/2(Executed) -> Switch/2
  input/1 -> Latch Input/1(Input)
  rising edge trigger/1 -> Latch Input/Trigger

== system Smart_City_QCar2_self_driving_stack_r2020a/QCar 2/QCar Control/QCar I//O ==
  note: '-w -d /tmp -uri %u', 'tcpip://192.168.1.3:17002'
  note: Command Conditioning
  note: HIL I/O
  note: LEDs:
      | 1. Back Left Amber
      | 2. Back Right Amber
      | 3. Front Left Amber
      | 4. Front Right Amber
      | 5. Brake Lights Red
      | 6. Reverse White
      | 7. Left Headlamps White
      | 8. Right Headlamps White
  "motorCmd (%, rad) [2]" : Inport
  Arm : Inport  Port=2
  Hazard : Inport  Port=3
  Volume : Inport  Port=4
  Honk : Inport  Port=5
  Abs : Abs
  Audio : Subsystem
  Constant1 : Constant
  Constant3 : Constant  Value=.05
  Constant4 : Constant  Value=.05
  Constant6 : Constant  Value=2
  Demux : Demux  Outputs=2
  Display : Display
  Gain : Gain  Gain=+1
  Greater Than Threshold : Subsystem
  HIL Initialize : quarc_library/Data Acquisition/Generic/Configuration/HIL Initialize  object_name=HIL-1  board_type=qcar2  board_number=0  board_options=gyro_fs=250;gyro_rate=500;gyro_bw=125;gyro_ord=3;accel_fs=16;accel_rate=1000;accel_bw=250;accel_ord=3;temp_bw=4000;enc0_dir=0;enc1_dir=0;enc2_dir=0;steer_bias=0.05;  exclusive=off  active=on  hardware_clocks=[]  clock_modes=[]  initial_clock_frequencies=[]  set_clock_params_at_start=off  set_clock_params_at_switch_in=off  set_clock_frequencies_at_start=off  set_clock_frequencies_at_switch_in=off  analog_input_channels=[0:4]  analog_input_configurations=[]  analog_input_maximums=[3.3]  analog_input_minimums=[0]  set_analog_input_params_at_start=off  set_analog_input_params_at_switch_in=off  analog_output_channels=[]  analog_output_maximums=[]  analog_output_minimums=[]  initial_analog_outputs=[]  final_analog_outputs=[]  watchdog_analog_outputs=[]  set_analog_output_params_at_start=off  set_analog_output_params_at_switch_in=off  set_analog_outputs_at_start=off  set_analog_outputs_at_switch_in=off  set_analog_outputs_at_terminate=off  set_analog_outputs_at_switch_out=off  set_analog_outputs_on_watchdog=off  digital_input_channels=[0:14]  digital_output_channels=[11:26]  digital_output_configuration=[]  initial_digital_outputs=[0]  final_digital_outputs=[0]  watchdog_digital_outputs=[0]  set_digital_output_params_at_start=off  set_digital_output_params_at_switch_in=off  set_digital_outputs_at_start=on  set_digital_outputs_at_switch_in=off  set_digital_outputs_at_terminate=on  set_digital_outputs_at_switch_out=off  set_digital_outputs_on_watchdog=off  encoder_channels=[0:2]  quadrature=[4]  encoder_filter_frequency=100e6/1  initial_encoder_counts=[0]  set_encoder_params_at_start=on  set_encoder_params_at_switch_in=off  set_encoder_counts_at_start=on  set_encoder_counts_at_switch_in=off  pwm_channels=[0:1]  pwm_modes=[0]  pwm_frequency=180e6/4096  pwm_configuration=[0]  pwm_alignment=[0]  pwm_polarity=[1]  pwm_leading_deadband=[]  pwm_trailing_deadband=[]  initial_pwm_outputs=[0]  final_pwm_outputs=[0]  watchdog_pwm_outputs=[0]  set_pwm_params_at_start=on  set_pwm_params_at_switch_in=off  set_pwm_outputs_at_start=on  set_pwm_outputs_at_switch_in=off  set_pwm_outputs_at_terminate=on  set_pwm_outputs_at_switch_out=off  set_pwm_outputs_on_watchdog=off  other_output_channels=[1000 11000]  initial_other_outputs=[0]  final_other_outputs=[0]  watchdog_other_outputs=[0]  set_other_outputs_at_start=on  set_other_outputs_at_switch_in=off  set_other_outputs_at_terminate=on  set_other_outputs_at_switch_out=off  set_other_outputs_on_watchdog=off
  HIL Read : quarc_library/Data Acquisition/Generic/Immediate I//O/HIL Read  object_name=HIL-1  analog_channels=[4 2]  encoder_channels=[0]  digital_channels=[]  other_channels=[14000 3002 4001]  sample_time=qc_get_step_size  active=on  vector_output=off  data_type_mode=Inherit via back propagation  encoder_data_type=double  digital_data_type=boolean
  HIL Write : quarc_library/Data Acquisition/Generic/Immediate I//O/HIL Write  object_name=HIL-1  analog_channels=[]  pwm_channels=[]  digital_channels=[17:18 25:26 11:16 19:24]  other_channels=[1000 11000]  sample_time=-1  active=off  vector_input=on
  LEDs : Subsystem
  Less Than Threshold1 : Subsystem
  MATLAB Function : MATLAB Function  TreatAsAtomicUnit=on
  Memory : Memory
  Mux : Mux  Inputs=2
  Scope : Scope
  Steering Bias : Bias  Bias=0.05*-1
  Unwrap 2^24 : quarc_library/Discontinuities/Inverse Modulus  modulus=16777215  output_derivative=off  output_revolutions=off  max_x=Inf  min_x=-Inf
  basicSpeedEstimation : Subsystem
  basicSpeedEstimation1 : Subsystem
  command saturation : Saturate  UpperLimit=.6  LowerLimit=-0.6
  direction convention : Gain  Gain=+1
  motorCurrent (A) [1] : Outport  VectorParamsAs1DForOutWhenUnconnected=off
  batteryVoltage (V) [1] : Outport  Port=2  VectorParamsAs1DForOutWhenUnconnected=off
  Speed (m/s) : Outport  Port=3  VectorParamsAs1DForOutWhenUnconnected=off
  gyroscopicRates (rad/s) : Outport  Port=4  VectorParamsAs1DForOutWhenUnconnected=off
  Odometer : Outport  Port=5  VectorParamsAs1DForOutWhenUnconnected=off
  wires:
  Demux/2 -> MATLAB Function/1(steering_in), LEDs/2(Steering)
  direction convention/1 -> command saturation/1
  "motorCmd (%, rad) [2]"/1 -> Demux/1
  HIL Read/3 -> Unwrap 2^24/1  "encoder counts"
  Gain/1 -> Steering Bias/1
  HIL Read/1 -> motorCurrent (A) [1]/1  "motor current"
  HIL Read/2 -> batteryVoltage (V) [1]/1  "battery voltage"
  HIL Read/4 -> basicSpeedEstimation/1(motorSpeed (counts/s))
  Unwrap 2^24/1 -> basicSpeedEstimation1/1(motorSpeed (counts/s))
  basicSpeedEstimation1/1(longitudinalCarSpeed (m/s)) -> Odometer/1
  basicSpeedEstimation/1(longitudinalCarSpeed (m/s)) -> [Speed], Speed (m/s)/1
  Demux/1 -> LEDs/1(Throttle), Scope/1, direction convention/1
  HIL Read/5 -> gyroscopicRates (rad/s)/1
  LEDs/1(LEDs) -> HIL Write/1
  Honk/1 -> Audio/1(Honk)
  Arm/1 -> Audio/2(Arm)
  [Speed] -> LEDs/3(Speed)
  Hazard/1 -> LEDs/4(Hazzard)
  HIL Read/6 -> Abs/1
  Abs/1 -> Greater Than Threshold/1(Signal)
  Constant6/1 -> Greater Than Threshold/2(Threshold)
  Constant1/1 -> Greater Than Threshold/3(Duration)
  Greater Than Threshold/1(elapsed) -> Audio/3(put_me_down)
  Volume/1 -> Audio/4(Volume)
  Constant3/1 -> Less Than Threshold1/2(Threshold)
  Constant4/1 -> Less Than Threshold1/3(Duration)
  [Speed] -> Less Than Threshold1/1(Signal)
  MATLAB Function/1(steering_out) -> Gain/1, Memory/1
  Less Than Threshold1/1(elapsed) -> Display/1, MATLAB Function/2(stopped)
  Memory/1 -> MATLAB Function/3(previous_steering)
  Mux/1 -> HIL Write/2
  Steering Bias/1 -> Mux/1
  command saturation/1 -> Mux/2

== system Smart_City_QCar2_self_driving_stack_r2020a/QCar 2/QCar Control/bicycleModel ==
  note: coordinate transformation
  note: Model side slip angle beta
  note: steering servo dynamics
  heading (rad) : Inport
  "motorCommands (%, rad)" : Inport  Port=2
  carSpeed (m/s) : Inport  Port=3
  gyroscope (rad/s) : Inport  Port=4
  Add : Sum
  Divide : Product  Inputs=*/
  Lr : Constant  Value=0.128
  Mux3 : Mux  Inputs=3
  Product : Product
  Product1 : Product
  Product2 : Product
  Transfer Fcn : TransferFcn  Denominator=[0.1026 1]
  Trigonometric Function : Trigonometry
  Trigonometric Function1 : Trigonometry  Operator=cos
  Trigonometric Function2 : Trigonometry  Operator=tan
  Trigonometric Function3 : Trigonometry  Operator=atan
  select steering : Selector  InputPortWidth=2  IndexOptions=Index vector (dialog)  Indices=[2]  OutputSizes=1
  steering servo dynamics : Scope  NumInputPorts=2
  wheelbase : Constant  Value=0.256
  "poseRate (m/s, m/s, rad/s)" : Outport  VectorParamsAs1DForOutWhenUnconnected=off
  wires:
  Add/1 -> Trigonometric Function1/1, Trigonometric Function/1
  Trigonometric Function1/1 -> Product1/2
  Product/1 -> Mux3/2  "y_dot"
  select steering/1 -> Transfer Fcn/1, steering servo dynamics/1  "delta"
  carSpeed (m/s)/1 -> Product/2, Product1/1  "v"
  Product1/1 -> Mux3/1  "x_dot"
  Trigonometric Function/1 -> Product/1
  gyroscope (rad/s)/1 -> Mux3/3  "psi_dot"
  heading (rad)/1 -> Add/1  "psi"
  "motorCommands (%, rad)"/1 -> select steering/1
  Mux3/1 -> "poseRate (m/s, m/s, rad/s)"/1
  Transfer Fcn/1 -> Trigonometric Function2/1, steering servo dynamics/2
  Divide/1 -> Trigonometric Function3/1
  wheelbase/1 -> Divide/2
  Product2/1 -> Divide/1  "Lr tan(delta)"
  Trigonometric Function3/1 -> Add/2  "beta"
  Trigonometric Function2/1 -> Product2/1  "tan(delta)"
  Lr/1 -> Product2/2  "Lr"

== system Smart_City_QCar2_self_driving_stack_r2020a/QCar 2/QCar Control/powerConsumptionMonitor ==
  note: Battery percentage calculation
  note: P = VI
  note: Electrical
      | power
      | consumed
  note: Power Monitoring Module:
      |
      | This subsystem monitors power consumption and provides a percentage battery remaining indicator.
      |
      | Inputs:
      | motorCurrent (A) n/a : Motor current being pulled by the main drive motor
      | batteryVoltage (V) {0, 12.6} : Current battery voltage reading
      |
      | Outputs:
      | motorPowerConsumption (W) n/a : Current power in Watts being pulled by the main drive motor
      | batteryLevel (%) {0,1} : Percentage battery level remaining
      |
      | Usage:
      | This is based on a maximum 3S battery voltage of 12.6 V (4.2V per cell) and minimum of 10.5 V (3.5V per cell)
  motorCurrent (A) [1] : Inport
  batteryVoltage (V) [1] : Inport  Port=2
  Divide : Product  Inputs=*/
  Gain : Gain  Gain=100
  Product : Product
  Subtract : Sum  Inputs=+-
  Subtract1 : Sum  Inputs=+-
  max voltage : Constant  Value=12.6
  min voltage : Constant  Value=10.5
  motorPowerConsumption (W) [1] : Outport  VectorParamsAs1DForOutWhenUnconnected=off
  batteryLevel (%) [1] : Outport  Port=2  VectorParamsAs1DForOutWhenUnconnected=off
  wires:
  Divide/1 -> Gain/1
  Subtract1/1 -> Divide/2
  Gain/1 -> batteryLevel (%) [1]/1
  Product/1 -> motorPowerConsumption (W) [1]/1
  min voltage/1 -> Subtract/2, Subtract1/2
  motorCurrent (A) [1]/1 -> Product/1
  max voltage/1 -> Subtract1/1
  Subtract/1 -> Divide/1
  batteryVoltage (V) [1]/1 -> Subtract/1, Product/2
